simulink model "final_2"  (R2024b)
settings: Solver=VariableStepAuto  StartTime=0.0  StopTime=10  RelTol=1e-3
undefined symbols (not defined in the file): dspblkCoreblockFVToolHelper, gcbh, Heso_sim
settings Model: Creator=Admin  LastModifiedBy=Admin

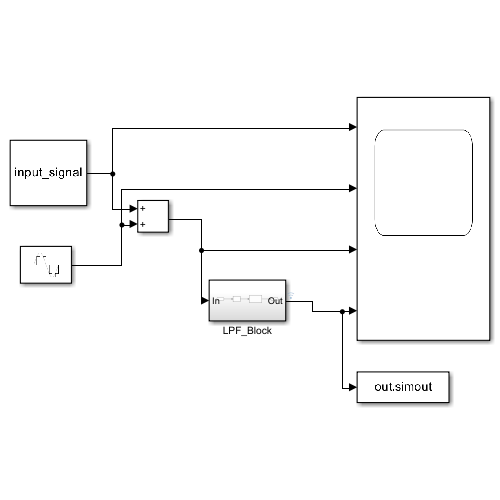
[thumbnail: Simulink's stored preview of the top-level diagram]
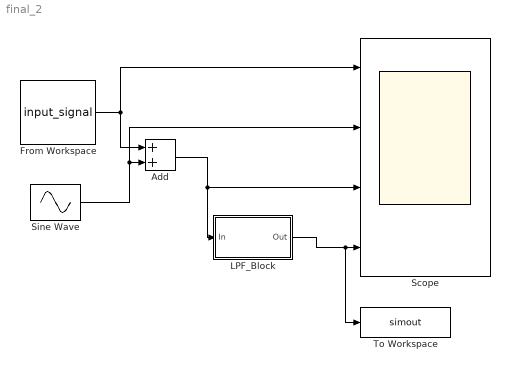
== system final_2 ==
  Add : Sum
  From Workspace : FromWorkspace  VariableName=input_signal  SampleTime=1/500  OutputAfterFinalValue=Holding final value
  LPF_Block : Subsystem  Tag=BlockMethodSubSystem
  Scope : Scope  NumInputPorts=4
  Sine Wave : Sin  Amplitude=0.5  Frequency=200*2*pi  SampleTime=1/500
  To Workspace : ToWorkspace  VariableName=simout  SampleTime=-1
  wires:
  Add/1 -> LPF_Block/1(In), Scope/3
  Sine Wave/1 -> Scope/2, Add/2
  From Workspace/1 -> Scope/1, Add/1
  LPF_Block/1(Out) -> To Workspace/1, Scope/4

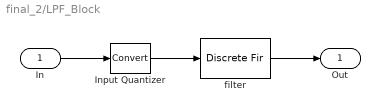
== system final_2/LPF_Block ==
  In : Inport
  Input Quantizer : DataTypeConversion  RndMeth=Round
  filter : DiscreteFir  LoadFcn=dspblkCoreblockFVToolHelper(gcbh,'load');  Coefficients=Heso_sim  InputProcessing=Columns as channels (frame based)  OutDataTypeStr=Inherit: Same as input
      settings: CopyFcn=dspblkCoreblockFVToolHelper(gcbh,'copy');  DeleteFcn=dspblkCoreblockFVToolHelper(gcbh,'close');  ModelCloseFcn=dspblkCoreblockFVToolHelper(gcbh,'close');  PreSaveFcn=dspblkCoreblockFVToolHelper(gcbh,'presave');  PostSaveFcn=dspblkCoreblockFVToolHelper(gcbh,'postsave');  CloseFcn=dspblkCoreblockFVToolHelper(gcbh,'close');
  Out : Outport
  wires:
  In/1 -> Input Quantizer/1
  Input Quantizer/1 -> filter/1
  filter/1 -> Out/1
